simulink model "HeartModelAll"  (R2014a)
settings: Solver=FixedStepDiscrete  StartTime=0.0  StopTime=100  FixedStep=0.01  RelTol=1e-3
undefined symbols (not defined in the file or in its folder): SA_d, T53_max, T53_mean, T53_min, T54_max, T54_mean, T54_min, T55_max, T55_mean, T55_min, T56_max, T56_mean, T56_min, T57_max, T57_mean, T57_min, T58_max, T58_mean, T58_min
settings Model: Creator=alexandru  LastModifiedBy=alexandru
settings DataIOCC: LimitDataPoints=off  SaveOutput=off  SignalLogging=off  DSMLogging=off  SaveTime=off
settings HardwareCC: TargetBitPerLong=64  TargetBitPerPointer=64  TargetLongLongMode=on  TargetIntDivRoundTo=Zero  TargetEndianess=LittleEndian  TargetWordSize=64  TargetHWDeviceType=MATLAB Host  ProdEqTarget=off
settings RTWCC: SystemTargetFile=rsim.tlc  GenCodeOnly=on  PackageGeneratedCodeAndArtifacts=on  PackageName=idhp_model_heart_realtime  TemplateMakefile=rsim_default_tmf  Description=Rapid Simulation Target  ProcessScript=rsim_make_rtw_hook
settings RSimTargetCC: ERTMultiwordTypeDef=System defined  ERTMultiwordLength=256  EnableShiftOperators=on

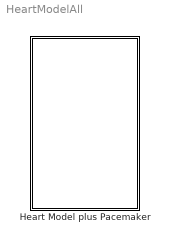
== system HeartModelAll ==
  Heart Model plus Pacemaker : Stateflow chart  Priority=1  TreatAsAtomicUnit=on

== stateflow chart HeartModelAll/Heart Model plus Pacemaker ==
  state Heart
    state A_dV [parallel]
      settings: executionOrder=13
      state a_dVLow
      state a_dvHigh
      (default) -> a_dVLow
      a_dVLow -> a_dvHigh [order 1] : a_dVSetHigh
      a_dVLow -> a_dVLow [order 2] : tr_AVJ
          | {send(AVJAnteReached,AVJ);}
      a_dvHigh -> a_dvHigh [order 2] : tr_AVJ
          | {send(AVJAnteReachedHigh,AVJ);}
      a_dvHigh -> a_dVLow [order 1] : a_dVSetLow
    state VtrNoiseGenerator [parallel]
      settings: executionOrder=3
      state q0
      (default) -> Heart.VtrNoiseGenerator.q0
      Heart.VtrNoiseGenerator.q0 -> Heart.VtrNoiseGenerator.q0 : after(VRG_noiseD, msec)
    state VRGEctopic [parallel]
      settings: executionOrder=10
      state q0
      (default) -> Heart.VRGEctopic.q0
      Heart.VRGEctopic.q0 -> Heart.VRGEctopic.q0 : after(VRG_ectopD, msec)
          | {send(Vbeat,Ventricle);}
    state RAConductor [parallel]
      settings: executionOrder=6
      state Empty
      state Ante
      state Retro
      (default) -> Heart.RAConductor.Empty
      Heart.RAConductor.Empty -> Heart.RAConductor.Ante [order 1] : arg
      Heart.RAConductor.Ante -> Heart.RAConductor.Empty [order 1] : retroAVJ
      Heart.RAConductor.Empty -> Heart.RAConductor.Retro [order 2] : retroAVJ
      Heart.RAConductor.Retro -> Heart.RAConductor.Empty [order 1] : arg
      Heart.RAConductor.Retro -> Heart.RAConductor.Empty [order 2] : after(RA_retroD,msec)
          | {send(AtrRetroReached,...
          | Atrium);}
      Heart.RAConductor.Ante -> Heart.RAConductor.Empty [order 2] : after(RA_anteD,msec)
          | {send(tr_AVJ,A_dV);}
    state AVJOut [parallel]
      settings: executionOrder=4
      state Empty
      state Ante
      state Retro
      (default) -> Heart.AVJOut.Empty
      Heart.AVJOut.Ante -> Heart.AVJOut.Empty : after(AVJDelay(avj_tRec,...
          | AV_anteDMin),msec)
          | {send(anteAVJ,RVConductor);}
      Heart.AVJOut.Empty -> Heart.AVJOut.Ante [order 1] : AVJAnteExit
      Heart.AVJOut.Retro -> Heart.AVJOut.Empty : after(AVJDelay(avj_tRec,...
          | AV_retroDMin),msec)
          | {send(retroAVJ,...
          | RAConductor);}
      Heart.AVJOut.Empty -> Heart.AVJOut.Retro [order 2] : AVJRetroExit
    state RVConductor [parallel]
      settings: executionOrder=5
      state Empty
      state Ante
      state Retro
      (default) -> Heart.RVConductor.Empty
      Heart.RVConductor.Empty -> Heart.RVConductor.Ante [order 1] : anteAVJ
      Heart.RVConductor.Empty -> Heart.RVConductor.Retro [order 2] : vrg
      Heart.RVConductor.Ante -> Heart.RVConductor.Empty [order 1] : vrg
      Heart.RVConductor.Ante -> Heart.RVConductor.Empty [order 2] : after(RV_anteD,msec)
          | {send(VtrAnteReached,...
          | Ventricle);}
      Heart.RVConductor.Retro -> Heart.RVConductor.Empty [order 1] : anteAVJ
      Heart.RVConductor.Retro -> Heart.RVConductor.Empty [order 2] : after(RV_retroD,msec)
          | {send(AVJRetroReached,...
          | AVJ);}
    state SANodeEctopic [parallel]
      settings: executionOrder=2
      state q0
      (default) -> Heart.SANodeEctopic.q0
      Heart.SANodeEctopic.q0 -> Heart.SANodeEctopic.q0 : after(SA_ectopD, msec)
          | {send(Abeat,Atrium);
          | send(a_dVSetHigh,A_dV);}
    state AtrNoiseGenerator [parallel]
      settings: executionOrder=1
      state q0
      Heart.AtrNoiseGenerator.q0 -> Heart.AtrNoiseGenerator.q0 : after(SA_noiseD, msec)
      (default) -> Heart.AtrNoiseGenerator.q0
    state VRG [parallel]
      settings: executionOrder=11
      state Wait4VBeat
      state Wait4VSynch
      (default) -> Wait4VBeat
      Wait4VBeat -> Wait4VSynch [order 2] : after(VRG_d, msec)
          | {send(Vbeat,Ventricle);}
      Wait4VSynch -> Wait4VBeat : NextVtrBeat
      Wait4VBeat -> Wait4VBeat [order 1] : NextVtrBeat
    state SANode [parallel]
      settings: executionOrder=7
      state Wait4ABeat
      state Wait4ASynch
      (default) -> Wait4ABeat
      Wait4ABeat -> Wait4ASynch [order 2] : after(SA_d, msec)
          | {send(Abeat,Atrium);
          | send(a_dVSetLow,A_dV);
          | }
      Wait4ABeat -> Wait4ABeat [order 1] : NextAtrBeat
      Wait4ASynch -> Wait4ABeat : NextAtrBeat
    state AVJ [parallel]
      settings: executionOrder=12
      state Recovery
      state Ante
      state Refractory
      state Retro
      Heart.AVJ.Ante -> Heart.AVJ.Refractory : after(avj_t4,msec)
          | {ctime=ctime+temporalCount(msec);
          | avj_tRec=(ctime-recoverylast);
          | send(AVJAnteExit,AVJOut);
          | avj_refr_0=initRefrPeriod(avj_tRec);
          | avj_refr=avj_refr_0;
          | refractorylast=ctime;}
      Recovery -> Heart.AVJ.Ante [order 1] : AVJAnteReached{
          | ctime=ctime+temporalCount(msec);
          | avj_t4 = timeToDep(AV_Vr+ ...
          | (ctime-recoverylast)*AV_k4 + SA_dV);
          | }
      Recovery -> Heart.AVJ.Ante [order 3] : AVJAnteReachedHigh{
          | ctime=ctime+temporalCount(msec);
          | avj_t4 = timeToDep(AV_Vr+...
          | (ctime-recoverylast)*AV_k4 + SA_ectopdV);
          | }
      Heart.AVJ.Refractory -> Recovery [order 4] : after(avj_refr,msec){
          | ctime=ctime+temporalCount(msec);
          | avj_t4=timeToDep(AV_Vr);
          | recoverylast=ctime;
          | }
      (default) -> Recovery : {
          | avj_t4=timeToDep(AV_Vr);
          | ctime=0;
          | recoverylast=0;
          | refractorylast=0;
          | }
      Recovery -> Heart.AVJ.Retro [order 4] : AVJRetroReached{
          | ctime=ctime+temporalCount(msec);}
      Recovery -> Heart.AVJ.Refractory [order 2] : after(avj_t4,msec){
          | ctime=ctime+temporalCount(msec);
          | avj_tRec=avj_t4;
          | avj_refr_0=initRefrPeriod(avj_tRec);
          | avj_refr=avj_refr_0;
          | refractorylast=ctime;}
      Heart.AVJ.Refractory -> Heart.AVJ.Refractory [order 3] : AVJAnteReachedHigh
          | {ctime=ctime+temporalCount(msec);
          | avj_refr=avj_refr-(ctime - refractorylast)+...
          | modulateRefrAnte((ctime - refractorylast),...
          | avj_refr_0,SA_ectopdV);
          | refractorylast=ctime;
          | }
      Heart.AVJ.Refractory -> Heart.AVJ.Refractory [order 1] : AVJAnteReached
          | {ctime=ctime+temporalCount(msec);
          | avj_refr=avj_refr-(ctime - refractorylast)+...
          | modulateRefrAnte((ctime - refractorylast),...
          | avj_refr_0,SA_dV);
          | refractorylast=ctime;}
      Heart.AVJ.Refractory -> Heart.AVJ.Refractory [order 2] : AVJRetroReached
          | {ctime=ctime+temporalCount(msec);
          | avj_refr=avj_refr-(ctime - refractorylast)+...
          | modulateRefrRetro((ctime - refractorylast),...
          | avj_refr_0);
          | refractorylast=ctime;}
      Heart.AVJ.Retro -> Heart.AVJ.Refractory : {send(AVJRetroExit,AVJOut);
          | ctime=ctime+temporalCount(msec);
          | avj_tRec=ctime-recoverylast;
          | avj_refr_0=initRefrPeriod(avj_tRec);
          | avj_refr=avj_refr_0;
          | refractorylast=ctime;
          | }
    state Ventricle [parallel]
      settings: executionOrder=8
      state Excitable
      state Refractory
      state VsenseAnte
      state VSynch
      state Vsense
      state GenerateRetroWave
      (default) -> Heart.Ventricle.Refractory
      Heart.Ventricle.Refractory -> Heart.Ventricle.Excitable : after(Vtr_refrD,msec)
      Heart.Ventricle.Excitable -> GenerateRetroWave [order 2] : VP
      Heart.Ventricle.Excitable -> Vsense [order 3] : Vbeat
      Heart.Ventricle.Excitable -> VsenseAnte [order 1] : VtrAnteReached
      VSynch -> Heart.Ventricle.Refractory : {send(NextVtrBeat,...
          | VRG);}
      VsenseAnte -> VSynch
      GenerateRetroWave -> VSynch : {send(vrg,RVConductor);}
      Vsense -> GenerateRetroWave
    state Atrium [parallel]
      settings: executionOrder=9
      state Excitable
      state Refractory
      state AsenseRetro
      state ASynch
      state Asense
      state GenerateAnteWave
      (default) -> Heart.Atrium.Refractory
      Heart.Atrium.Excitable -> Asense [order 1] : Abeat
      Heart.Atrium.Refractory -> Heart.Atrium.Excitable : after(Atr_refrD,msec)
      Heart.Atrium.Excitable -> AsenseRetro [order 3] : AtrRetroReached
      ASynch -> Heart.Atrium.Refractory : {send(NextAtrBeat,...
          | SANode);}
      Heart.Atrium.Excitable -> GenerateAnteWave [order 2] : AP
      AsenseRetro -> ASynch
      GenerateAnteWave -> ASynch : {send(arg,RAConductor);}
      Asense -> GenerateAnteWave
    state VRP [parallel]
      settings: executionOrder=18
      state Idle
      state VRP
      state Vsig
      Heart.VRP.VRP -> Heart.VRP.Idle : after(PM_TVRP,msec)
        settings: description=|
            | Cosmos
            | T56
      (default) -> Heart.VRP.Idle
      Heart.VRP.Idle -> Heart.VRP.VRP [order 2] : VP
      Vsig -> Heart.VRP.Idle : {send(RLRI, LRI);
          | send(VS, AVI);
          | send(VS, PVARP);}
      Heart.VRP.Idle -> Vsig [order 1] : Vget
    state LRI [parallel]
      settings: executionOrder=14
      state LRI
      state ASensed
      Heart.LRI.LRI -> Heart.LRI.LRI [order 2] : after(PM_TLRI-PM_TAVI,msec)
          | {send(AP,AVI);send(AP,Atrium);}
        settings: description=|
            | Cosmos
            | T53
      Heart.LRI.LRI -> ASensed [order 3] : AS
      ASensed -> Heart.LRI.LRI : RLRI
      Heart.LRI.LRI -> Heart.LRI.LRI [order 1] : RLRI
      (default) -> Heart.LRI.LRI
    state URI [parallel]
      settings: executionOrder=15
      state URI
      state q1
      Heart.URI.URI -> Heart.URI.URI [order 1] : RURI
      (default) -> Heart.URI.URI
      Heart.URI.URI -> Heart.URI.q1 [order 2] : after(PM_TURI,msec)
          | {send(IncrClk,AVI);}
        settings: description=|
            | Cosmos
            | T54
      Heart.URI.q1 -> Heart.URI.URI
    state AVI [parallel]
      settings: executionOrder=17
      state Idle0
      state AVI0
      state WaitURI
      state Idle1
      state AVI1
      WaitURI -> Idle0 [order 1] : VS{send(RURI,URI);}
      AVI0 -> Idle0 [order 3] : VS{send(RURI,URI);}
      Idle0 -> AVI0 [order 2] : AP{send(RTAVI,TAVIcmp);}
      (default) -> Idle0
      AVI0 -> WaitURI [order 2] : TAVI
      Idle0 -> AVI0 [order 3] : AS{send(RTAVI,TAVIcmp);}
      AVI1 -> Idle0 [order 2] : TAVI{
          | send(RLRI,LRI);
          | send(VP,VRP);
          | send(VP,PVARP);
          | send(RURI,URI);
          | send(VP,Ventricle);}
      AVI1 -> Idle0 [order 1] : VS{send(RURI,URI);}
      WaitURI -> Idle0 [order 2] : IncrClk{
          | send(RLRI,LRI);
          | send(VP,VRP);
          | send(VP,PVARP);
          | send(VP,Ventricle);}
      AVI0 -> AVI1 [order 1] : IncrClk
      Idle0 -> Idle1 [order 1] : IncrClk
      Idle1 -> AVI1 [order 2] : AP{send(RTAVI,TAVIcmp);}
      Idle1 -> AVI1 [order 1] : AS{send(RTAVI,TAVIcmp);}
    state TAVIcmp [parallel]
      settings: executionOrder=16
      state q0
      state q1
      Heart.TAVIcmp.q0 -> Heart.TAVIcmp.q1 : after(PM_TAVI,msec)
          | {send(TAVI,AVI);}
        settings: description=|
            | Cosmos
            | T55
      Heart.TAVIcmp.q1 -> Heart.TAVIcmp.q0 : RTAVI
      (default) -> Heart.TAVIcmp.q1
    state PVARP [parallel]
      settings: executionOrder=19
      state Idle
      state PVAB
      state Asig
      state PVARP
      Heart.PVARP.Idle -> PVAB [order 3] : VP
      Heart.PVARP.Idle -> PVAB [order 2] : VS
      (default) -> Heart.PVARP.Idle
      Heart.PVARP.PVARP -> Heart.PVARP.Idle : after(PM_TPVARP-...
          | PM_TPVAB,msec)
        settings: description=|
            | Cosmos
            | T57
      Asig -> Heart.PVARP.Idle : {send(AS,LRI);
          | send(AS,AVI);
          | send(AS,TAVIcmp);}
      Heart.PVARP.Idle -> Asig [order 1] : Aget
      PVAB -> Heart.PVARP.PVARP : after(PM_TPVAB,msec)
        settings: description=|
            | Cosmos
            | T58
    state InitBatt [parallel]
      settings: executionOrder=20
      state Init
      (default) -> Init : {ResetBatteryState();}
  (default) -> Heart
  data: t function_output double; tRec function_input double; minDly function_input double; t function_output double; Vm function_input double; t function_input double; t0 function_input double; dT function_output double; dV function_input double; t function_input double; dT function_output double; t0 function_input double; t function_output double; tRec function_input double; Atr_refrD local double =50; AV_alpha local double =150; AV_anteDMin local double =50; AV_beta local double =250; AV_delta local double =10; AV_k4 local double =0.03; AV_refrDMin local double =50; AV_retroDMin local double =100; AV_tauC local double =100; AV_theta local double =10; AV_tr local double =500; AV_Vr local double =-90; AV_Vt local double =-40; RA_anteD local double =30; RA_retroD local double =30; RV_anteD local double =50; RV_retroD local double =50; SA_d parameter double =1000; SA_dV local double =50; SA_ectopD local double =10400; SA_ectopdV local double =50; SA_noiseD local double =1000000; VRG_d local double =3000; VRG_ectopD local double =30450; VRG_noiseD local double =1000000; Vtr_refrD local double =200; avj_tRec local double; clk local double; recoverylast local double; avj_t4 local double; ctime local double; avj_refr local double; avj_refr_0 local double; refractorylast local double; BAUDRATE local uint32 =57600; bufs1 local uint8; bufs2 local uint8; bufs3 local uint8; bufs4 local uint8; bufs5 local uint8; parid local uint16; value local uint32; parval local double; tmp16 local uint16; tmp32 local uint32; PM_TAVI local uint32 =131; PM_TPVAB local uint32 =50; PM_TPVARP local uint32 =250; PM_TURI local uint32 =500; PM_TVRP local uint32 =320; PM_TLRI local uint32 =1000; T53_min parameter double; T53_max parameter double; T53_mean parameter double; T54_min parameter double; T54_max parameter double; T54_mean parameter double; T55_mean parameter double; T56_mean parameter double; T57_mean parameter double; T58_mean parameter double; T55_min parameter double; T56_min parameter double; T57_min parameter double; T58_min parameter double; T55_max parameter double; T56_max parameter double; T57_max parameter double; T58_max parameter double
  events: Abeat local FUNCTION_CALL_EVENT; AtrRetroReached local FUNCTION_CALL_EVENT; arg local FUNCTION_CALL_EVENT; retroAVJ local FUNCTION_CALL_EVENT; AVJAnteReached local FUNCTION_CALL_EVENT; NextAtrBeat local FUNCTION_CALL_EVENT; AVJRetroReached local FUNCTION_CALL_EVENT; anteAVJ local FUNCTION_CALL_EVENT; vrg local FUNCTION_CALL_EVENT; VtrAnteReached local FUNCTION_CALL_EVENT; AVJRetroExit local FUNCTION_CALL_EVENT; AVJAnteExit local FUNCTION_CALL_EVENT; NextVtrBeat local FUNCTION_CALL_EVENT; Vbeat local FUNCTION_CALL_EVENT; AP local EITHER_EDGE_EVENT; VP local EITHER_EDGE_EVENT; AS local RISING_EDGE_EVENT; VS local RISING_EDGE_EVENT; Aget local EITHER_EDGE_EVENT; Vget local EITHER_EDGE_EVENT; Aintrinsic local EITHER_EDGE_EVENT; Anoise local EITHER_EDGE_EVENT; Aretro local EITHER_EDGE_EVENT; Vintrinsic local EITHER_EDGE_EVENT; Vnoise local EITHER_EDGE_EVENT; APElectr local RISING_EDGE_EVENT; VPElectr local EITHER_EDGE_EVENT; IncrClk local FUNCTION_CALL_EVENT; State local FUNCTION_CALL_EVENT; Clk0 local FUNCTION_CALL_EVENT; Clk1 local FUNCTION_CALL_EVENT; a_dVSetHigh local FUNCTION_CALL_EVENT; a_dVSetLow local FUNCTION_CALL_EVENT; tr_AVJ local FUNCTION_CALL_EVENT; AVJAnteReachedHigh local FUNCTION_CALL_EVENT; RLRI local FUNCTION_CALL_EVENT; TAVI local FUNCTION_CALL_EVENT; RTAVI local FUNCTION_CALL_EVENT; RURI local FUNCTION_CALL_EVENT
  function t  = AVJDelay(tRec,minDly):
    | function t  = AVJDelay(tRec,minDly)
    |     t = minDly+AV_alpha*exp(-tRec/AV_tauC);
    | end
  function t  = timeToDep(Vm):
    | function t  = timeToDep(Vm)
    |     t = max(0,(AV_Vt-Vm)/AV_k4);
    | end
  function dT  = modulateRefrAnte(t,t0,dV):
    | function dT  = modulateRefrAnte(t,t0,dV)
    |     %val1 = t/t0;
    |     %val2 = power(t/t0,avj_theta);
    |     dT = AV_refrDMin*power(t/t0,AV_theta)*power(min(1,dV/(AV_Vt-AV_Vr)),AV_delta);
    |     %fprintf(1,'%f %f\n', val1, val2);
    | end
  function dT  = modulateRefrRetro(t,t0):
    | 
    | function dT  = modulateRefrRetro(t,t0)
    |     dT = AV_refrDMin*power(t/t0,AV_theta);
    | end
  function t  = initRefrPeriod(tRec):
    | function t  = initRefrPeriod(tRec)
    |     t = AV_refrDMin + AV_beta*(1 - exp(-tRec/AV_tr));
    | end
